simulink model "simulink_01_linearizzatp"  (R2024b)
settings: Solver=VariableStepAuto  StartTime=0.0  StopTime=1.0  RelTol=1e-3
values from neighbouring files (symbols this model uses):
  alpha_0 = invpendulumP.alpha_0    [CODE_42_01.m]    (also in nonlinear_analisys_and_simulation.m)
  alpha_1 = invpendulumP.alpha_1    [CODE_42_01.m]    (also in nonlinear_analisys_and_simulation.m)
  b = invpendulumP.b    [CODE_42_01.m]    (also in nonlinear_analisys_and_simulation.m = 0)
  c = invpendulumP.c    [CODE_42_01.m]    (also in nonlinear_analisys_and_simulation.m = 0)
  g = invpendulumP.g    [CODE_42_01.m]    (also in nonlinear_analisys_and_simulation.m)
  I_0 = invpendulumP.I_0    [CODE_42_01.m]    (also in nonlinear_analisys_and_simulation.m)
  I_1 = invpendulumP.I_1    [CODE_42_01.m]    (also in nonlinear_analisys_and_simulation.m)
  I_2 = invpendulumP.I_2    [CODE_42_01.m]    (also in nonlinear_analisys_and_simulation.m)
  M = invpendulumP.M    [CODE_42_01.m]    (also in nonlinear_analisys_and_simulation.m)
settings Model: Creator=palla  LastModifiedBy=palla

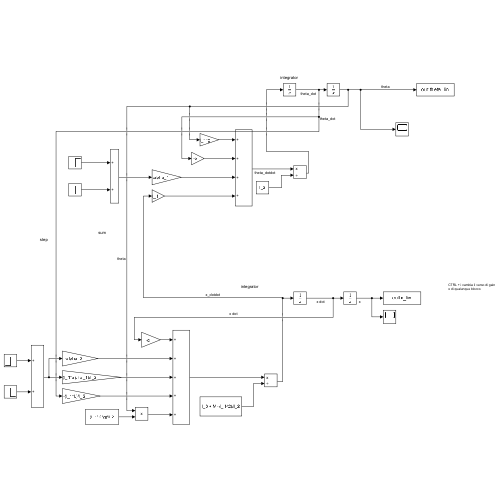
[thumbnail: Simulink's stored preview of the top-level diagram]
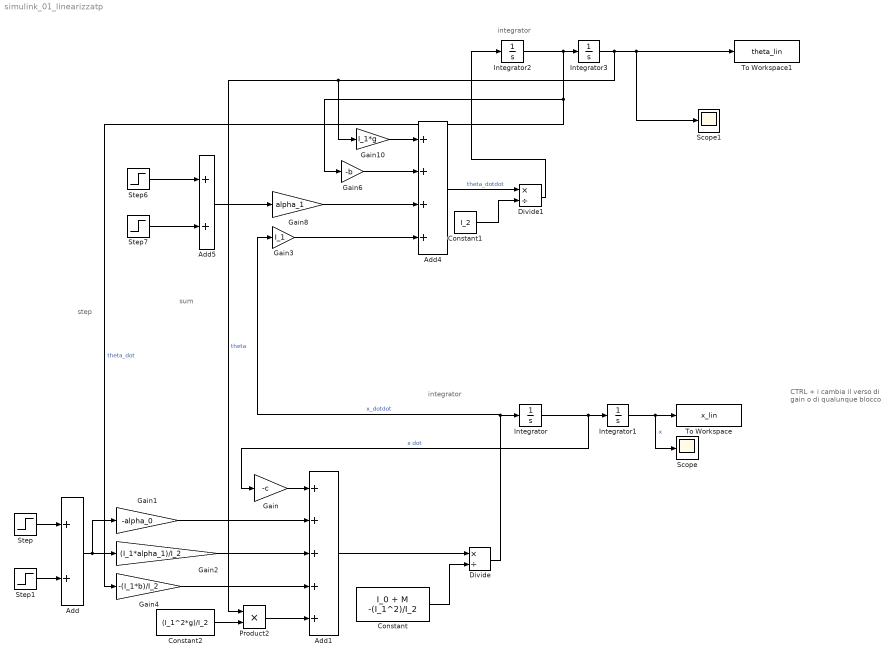
== system simulink_01_linearizzatp ==
  note: integrator
  note: sum
  note: integrator
  note: CTRL + i cambia il verso di gain
      | o di qualunque blocco
  note: step
  Add : Sum
  Add1 : Sum  Inputs=+++++
  Add4 : Sum  Inputs=++++
  Add5 : Sum
  Constant : Constant  Value=I_0 + M -(I_1^2)/I_2
  Constant1 : Constant  Value=I_2
  Constant2 : Constant  Value=(I_1^2*g)/I_2
  Divide : Product  Inputs=*/
  Divide1 : Product  Inputs=*/
  Gain : Gain  Gain=-c
  Gain1 : Gain  Gain=-alpha_0
  Gain10 : Gain  Gain=I_1*g
  Gain2 : Gain  Gain=(I_1*alpha_1)/I_2
  Gain3 : Gain  Gain=I_1
  Gain4 : Gain  Gain=-(I_1*b)/I_2
  Gain6 : Gain  Gain=-b
  Gain8 : Gain  Gain=alpha_1
  Integrator{,1..3} (4 alike) : Integrator
  Product2 : Product
  Scope : Scope
  Scope1 : Scope
  Step : Step  SampleTime=0
  Step1 : Step  Time=3  After=-1  SampleTime=0
  Step6 : Step  SampleTime=0
  Step7 : Step  Time=3  After=-1  SampleTime=0
  To Workspace : ToWorkspace  VariableName=x_lin  SampleTime=-1
  To Workspace1 : ToWorkspace  VariableName=theta_lin  SampleTime=-1
  wires:
  Constant1/1 -> Divide1/2
  Add1/1 -> Divide/1
  Gain3/1 -> Add4/4
  Gain/1 -> Add1/1
  Constant2/1 -> Product2/2
  Integrator2/1 -> Gain6/1, Gain4/1, Integrator3/1  "theta_dot"
  Gain1/1 -> Add1/2
  Divide1/1 -> Integrator2/1
  Integrator/1 -> Gain/1, Integrator1/1  "x dot"
  Integrator1/1 -> To Workspace/1, Scope/1  "x"
  Step6/1 -> Add5/1
  Integrator3/1 -> Gain10/1, Product2/1, Scope1/1, To Workspace1/1  "theta"
  Add4/1 -> Divide1/1  "theta_dotdot"
  Add/1 -> Gain1/1, Gain2/1
  Add5/1 -> Gain8/1
  Gain8/1 -> Add4/3
  Step/1 -> Add/1
  Product2/1 -> Add1/5
  Gain4/1 -> Add1/4
  Gain6/1 -> Add4/2
  Gain10/1 -> Add4/1
  Divide/1 -> Gain3/1, Integrator/1  "x_dotdot"
  Gain2/1 -> Add1/3
  Step1/1 -> Add/2
  Constant/1 -> Divide/2
  Step7/1 -> Add5/2
